simulink model "Bouc_wen_model"  (R2019a)
settings: Solver=ode45  StartTime=0.0  StopTime=5  MaxStep=0.001  MinStep=0.000005  RelTol=1e-3
values from neighbouring files (symbols this model uses):
  A = 301    [Bouc_wen_paper.m]
  alph_a = 140    [Bouc_wen_paper.m]
  alph_b = 695    [Bouc_wen_paper.m]
  Amp = 1.5    [Bouc_wen_paper.m]
  bta = gam    (= 363)    [Bouc_wen_paper.m]
  c0a = 21    [Bouc_wen_paper.m]
  c0b = 3.5    [Bouc_wen_paper.m]
  c1a = 283    [Bouc_wen_paper.m]
  c1b = 2.95    [Bouc_wen_paper.m]
  eta = 190    [Bouc_wen_paper.m]
  freq_ = 3*pi    (= 9.42477796077)    [Bouc_wen_paper.m]
  gam = 363    [Bouc_wen_paper.m]
  k0 = 46.9    [Bouc_wen_paper.m]
  k1 = 5    [Bouc_wen_paper.m]
  n = 2    [Bouc_wen_paper.m]
  phase_ = -pi/2    (= -1.57079632679)    [Bouc_wen_paper.m]
  V = 3    [Bouc_wen_paper.m]
  x0 = 14.3    [Bouc_wen_paper.m]
settings Model: Creator=Jose Sosa  LastModifiedBy=Jose Sosa
settings SolverCC: InitialStep=0.0001  ZeroCrossAlgorithm=Adaptive
settings DataIOCC: ReturnWorkspaceOutputs=off
settings OptimizationCC: LifeSpan=inf
settings DebuggingCC: SFExecutionAtInitializationDiag=none  ArithmeticOperatorsInVariantConditions=warning
settings HardwareCC: ProdBitPerSizeT=32  ProdBitPerPtrDiffT=32  ProdWordSize=32  ProdHWDeviceType=Specified
settings CodeAppCC: StateflowObjectComments=on

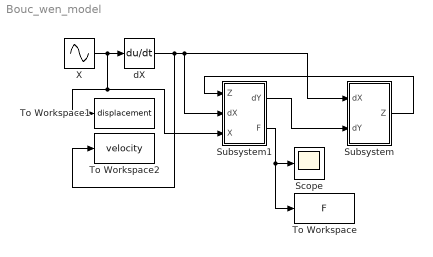
== system Bouc_wen_model ==
  Scope : Scope
  Subsystem : Subsystem
  Subsystem1 : Subsystem
  To Workspace : ToWorkspace  VariableName=F  SampleTime=-1
  To Workspace1 : ToWorkspace  VariableName=displacement  SampleTime=-1
  To Workspace2 : ToWorkspace  VariableName=velocity  SampleTime=-1
  X : Sin  Amplitude=Amp  Frequency=freq_  Phase=phase_  SampleTime=0
  dX : Derivative
  wires:
  Subsystem1/1(dY) -> Subsystem/2(dY)
  Subsystem/1(Z) -> Subsystem1/1(Z)
  dX/1 -> To Workspace2/1, Subsystem1/2(dX), Subsystem/1(dX)
  X/1 -> Subsystem1/3(X), To Workspace1/1, dX/1
  Subsystem1/2(F) -> To Workspace/1, Scope/1

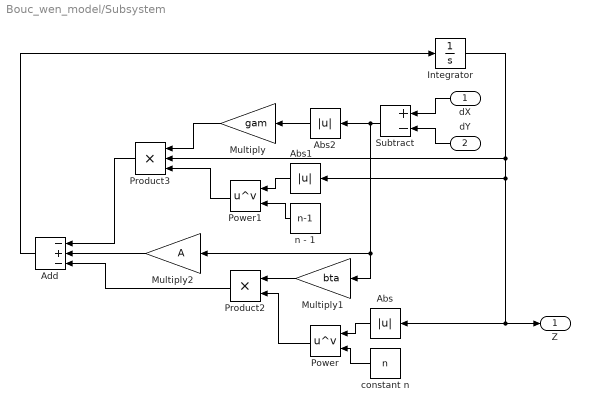
== system Bouc_wen_model/Subsystem ==
  dX : Inport
  dY : Inport  Port=2
  Abs : Abs
  Abs1 : Abs
  Abs2 : Abs
  Add : Sum  Inputs=-+-
  Integrator : Integrator
  Multiply : Gain  Gain=gam
  Multiply1 : Gain  Gain=bta
  Multiply2 : Gain  Gain=A
  Power : Math  Operator=pow  SaturateOnIntegerOverflow=on
  Power1 : Math  Operator=pow  SaturateOnIntegerOverflow=on
  Product2 : Product
  Product3 : Product  Inputs=3
  Subtract : Sum  Inputs=+-
  constant n : Constant  Value=n
  n - 1 : Constant  Value=n-1
  Z : Outport
  wires:
  Subtract/1 -> Multiply1/1, Multiply2/1, Abs2/1
  dX/1 -> Subtract/1
  Abs1/1 -> Power1/1
  Integrator/1 -> Product3/2, Z/1, Abs/1, Abs1/1
  constant n/1 -> Power/2
  Abs/1 -> Power/1
  n - 1/1 -> Power1/2
  Multiply/1 -> Product3/1
  dY/1 -> Subtract/2
  Power/1 -> Product2/2
  Abs2/1 -> Multiply/1
  Product3/1 -> Add/1
  Add/1 -> Integrator/1
  Power1/1 -> Product3/3
  Multiply1/1 -> Product2/1
  Product2/1 -> Add/3
  Multiply2/1 -> Add/2

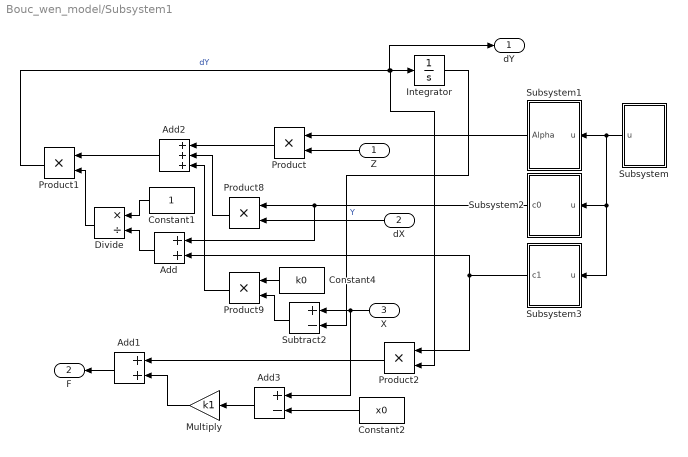
== system Bouc_wen_model/Subsystem1 ==
  Z : Inport
  dX : Inport  Port=2
  X : Inport  Port=3
  Add : Sum
  Add1 : Sum
  Add2 : Sum  Inputs=+++
  Add3 : Sum  Inputs=+-
  Constant1 : Constant
  Constant2 : Constant  Value=x0
  Constant4 : Constant  Value=k0
  Divide : Product  Inputs=*/
  Integrator : Integrator
  Multiply : Gain  Gain=k1
  Product{,1..2,8..9} (5 alike) : Product
  Subsystem : Subsystem
  Subsystem1 : Subsystem
  Subsystem2 : Subsystem
  Subsystem3 : Subsystem
  Subtract2 : Sum  Inputs=+-
  dY : Outport
  F : Outport  Port=2
  wires:
  dX/1 -> Product8/2
  Subtract2/1 -> Product9/2
  Product9/1 -> Add2/3
  Subsystem1/1(Alpha) -> Product/1
  Integrator/1 -> Subtract2/2  "Y"
  Product8/1 -> Add2/2
  Constant4/1 -> Product9/1
  Subsystem2/1(c0) -> Add/1, Product8/1
  X/1 -> Add3/1, Subtract2/1
  Product/1 -> Add2/1
  Add2/1 -> Product1/1
  Z/1 -> Product/2
  Subsystem/1(u) -> Subsystem3/1(u), Subsystem2/1(u), Subsystem1/1(u)
  Add/1 -> Divide/2
  Constant1/1 -> Divide/1
  Divide/1 -> Product1/2
  Product1/1 -> dY/1, Product2/2, Integrator/1  "dY"
  Subsystem3/1(c1) -> Product2/1, Add/2
  Product2/1 -> Add1/1
  Constant2/1 -> Add3/2
  Add3/1 -> Multiply/1
  Multiply/1 -> Add1/2
  Add1/1 -> F/1

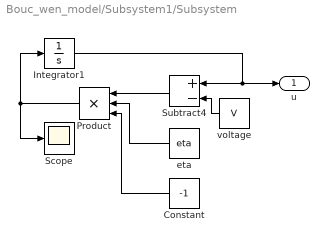
== system Bouc_wen_model/Subsystem1/Subsystem ==
  Constant : Constant  Value=-1
  Integrator1 : Integrator
  Product : Product  Inputs=3
  "Scope " : Scope
  Subtract4 : Sum  Inputs=+-
  eta : Constant  Value=eta
  voltage : Constant  Value=V
  u : Outport
  wires:
  Subtract4/1 -> Product/1
  Integrator1/1 -> Subtract4/1, u/1
  voltage/1 -> Subtract4/2
  eta/1 -> Product/2
  Constant/1 -> Product/3
  Product/1 -> Integrator1/1, "Scope "/1

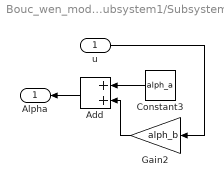
== system Bouc_wen_model/Subsystem1/Subsystem1 ==
  u : Inport
  Add : Sum
  Constant3 : Constant  Value=alph_a
  Gain2 : Gain  Gain=alph_b
  Alpha : Outport
  wires:
  Gain2/1 -> Add/2
  u/1 -> Gain2/1
  Add/1 -> Alpha/1
  Constant3/1 -> Add/1

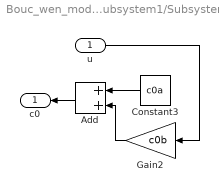
== system Bouc_wen_model/Subsystem1/Subsystem2 ==
  u : Inport
  Add : Sum
  Constant3 : Constant  Value=c0a
  Gain2 : Gain  Gain=c0b
  c0 : Outport
  wires:
  u/1 -> Gain2/1
  Add/1 -> c0/1
  Constant3/1 -> Add/1
  Gain2/1 -> Add/2

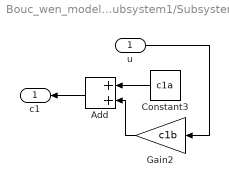
== system Bouc_wen_model/Subsystem1/Subsystem3 ==
  u : Inport
  Add : Sum
  Constant3 : Constant  Value=c1a
  Gain2 : Gain  Gain=c1b
  c1 : Outport
  wires:
  Add/1 -> c1/1
  Gain2/1 -> Add/2
  Constant3/1 -> Add/1
  u/1 -> Gain2/1
